simulink model "Piccolo_Induction_Motor(2)"  (R2022b)
settings: Solver=ode1  StartTime=0.0  StopTime=Inf  FixedStep=0.0001  RelTol=1e-3  EnableMultiTasking=on
PostLoadFcn:
  | ,try, rti_mdl_postloadfcn(bdroot, 'UpdateModel', 320, 'rti1104'); catch, disp(lasterr); end,
undefined symbols (not defined in the file or in its folder): Down, GPTRIP1SEL, GPTRIP2SEL, Km, TZ1, TZ2, Up
libraries: c2802xlib x3, c2806xlib x2, simulink x1, rtilib1104 x1, Piccolo_Library x1, c280xlib x1
settings Model: ExtModeTrigDuration=8  Creator=sb35user  LastModifiedBy=carls
settings SolverCC: ZeroCrossAlgorithm=Non-adaptive  AlgebraicLoopSolver=TrustRegion
settings DataIOCC: LimitDataPoints=on  SaveFormat=Array  SignalLoggingSaveFormat=ModelDataLogs  ReturnWorkspaceOutputs=off
settings OptimizationCC: BlockReduction=off  DefaultUnderspecifiedDataType=single  EnhancedBackFolding=on  PassReuseOutputArgsAs=Individual arguments  ExpressionDepthLimit=2147483647  InitFltsAndDblsToZero=on  MaxStackSize=1024  OptimizeBlockOrder=speed  DifferentSizesBufferReuse=on  OptimizationCustomize=off  DenormalBehavior=FlushToZero  EfficientTunableParamExpr=on
settings DebuggingCC: UnderspecifiedInitializationDetection=Classic  MergeDetectMultiDrivingBlocksExec=none  SolverPrmCheckMsg=warning  ParameterTunabilityLossMsg=error  FcnCallInpInsideContextMsg=warning  UnconnectedInputMsg=warning  UnconnectedOutputMsg=warning  UnconnectedLineMsg=warning  StateNameClashWarn=warning  SFUnexpectedBacktrackingDiag=warning  SFNoUnconditionalDefaultTransitionDiag=warning  SFExecutionAtInitializationDiag=none  SFMachineParentedDataDiag=warning  ArithmeticOperatorsInVariantConditions=warning
settings HardwareCC: ProdBitPerChar=16  ProdBitPerInt=16  ProdBitPerPointer=32  ProdBitPerSizeT=32  ProdBitPerPtrDiffT=32  ProdLargestAtomicInteger=Integer  ProdLargestAtomicFloat=None  ProdWordSize=16  ProdLongLongMode=on  ProdHWDeviceType=Texas Instruments->C2000  TargetIntDivRoundTo=Zero  TargetEndianess=BigEndian
settings ModelReferenceCC: PropagateSignalLabelsOutOfModel=off
settings SFSimCC: MATLABDynamicMemAlloc=off
settings RTWCC: Description=Embedded Coder  SystemTargetFile=ert.tlc  HardwareBoard=TI Piccolo F28069M LaunchPad  TLCOptions=-aInlineSetEventsForThisBaseRateFcn=TLC_FALSE -aSuppressMultiTaskScheduler=TLC_FALSE -aRateBasedStepFcn=1  TemplateMakefile=ert_default_tmf  Toolchain=Texas Instruments Code Composer Studio (C2000)
settings CodeAppCC: ForceParamTrailComments=on  IgnoreCustomStorageClasses=off  OperatorAnnotations=on  SimulinkDataObjDesc=on  SFDataObjDesc=on  InsertBlockDesc=on
settings ERTTargetCC: CodeReplacementLibrary=TI C28x  SupportContinuousTime=on  ExtModeTransport=4  ExtModeStaticAlloc=on  ExtModeAutomaticAllocSize=off  ExtModeMexFile=ext_xcp  ExtModeIntrfLevel=Level2 - Open
settings ConfigComp: CovMetricSettings=dw  CovSaveCumulativeToWorkspaceVar=on  CovSaveSingleToWorkspaceVar=on

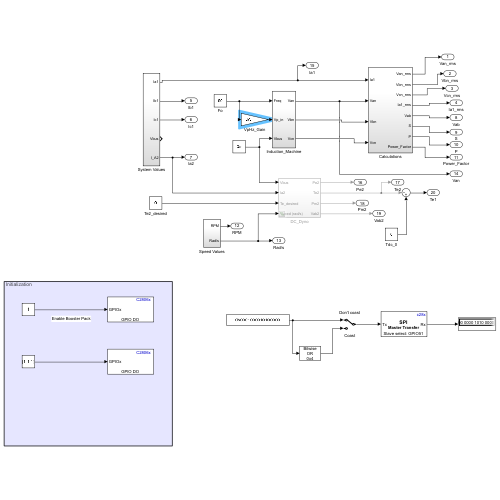
[thumbnail: Simulink's stored preview of the top-level diagram]
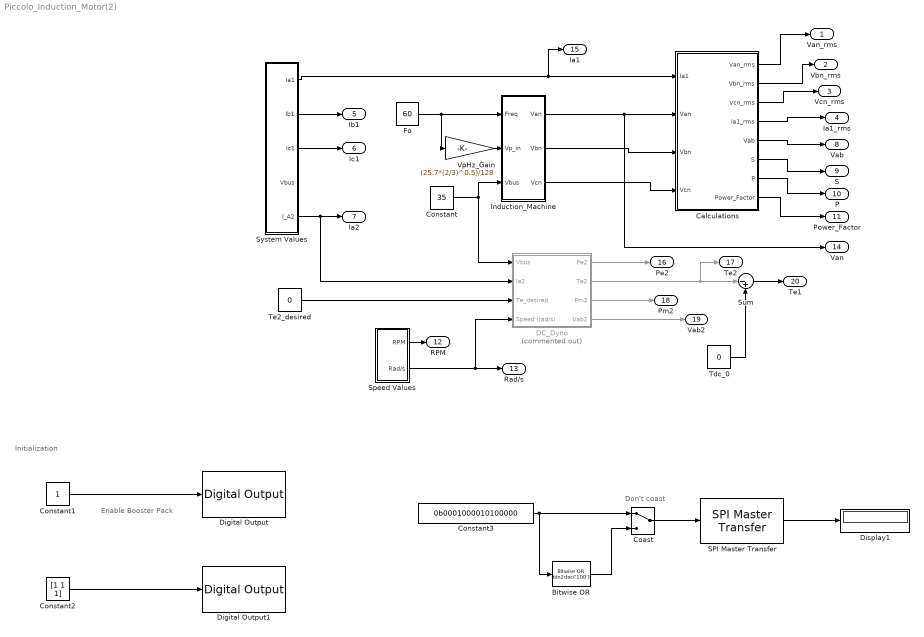
== system Piccolo_Induction_Motor(2) ==
  note: Don't coast
  note: Enable Booster Pack
  note: Initialization
  Bitwise OR : simulink/Logic and Bit Operations/Bitwise Operator  logicop=OR  UseBitMask=on  BitMask=bin2dec('100')  BitMaskRealWorld=Stored Integer
      settings: LibrarySourceBlock=|
      | simulink/Quick Insert/Logic and Bit
      | Operations/Bitwise OR
  Calculations : Subsystem
  Coast : ManualSwitch
  Constant : Constant  Value=35
  Constant1 : Constant
  Constant2 : Constant  Value=[1 1 1]
  Constant3 : Constant  Value=0b0001000010100000
  DC_Dyno : Subsystem  Commented=on
  Digital Output : c2806xlib/Digital Output  GPIO_Number=GPIO8~GPIO15  GPIO_Bit0=off  GPIO_BIT0_Toggle=off  GPIO_Bit1=off  GPIO_BIT1_Toggle=off  GPIO_Bit2=off  GPIO_BIT2_Toggle=off  GPIO_Bit3=off  GPIO_BIT3_Toggle=off  GPIO_Bit4=on  GPIO_BIT4_Toggle=off  GPIO_Bit5=off  GPIO_BIT5_Toggle=off  GPIO_Bit6=off  GPIO_BIT6_Toggle=off  GPIO_Bit7=off  GPIO_BIT7_Toggle=off
  Digital Output1 : c2806xlib/Digital Output  GPIO_Number=GPIO0~GPIO7  GPIO_Bit0=off  GPIO_BIT0_Toggle=off  GPIO_Bit1=on  GPIO_BIT1_Toggle=off  GPIO_Bit2=off  GPIO_BIT2_Toggle=off  GPIO_Bit3=on  GPIO_BIT3_Toggle=off  GPIO_Bit4=off  GPIO_BIT4_Toggle=off  GPIO_Bit5=on  GPIO_BIT5_Toggle=off  GPIO_Bit6=off  GPIO_BIT6_Toggle=off  GPIO_Bit7=off  GPIO_BIT7_Toggle=off
  Display1 : Display
      settings: Format=binary (Stored Integer)
  Fo : Constant  Value=60
  Induction_Machine : Subsystem
  SPI Master Transfer : c280xlib/SPI Master Transfer  SPISelect=SPI_A  ClockPolarity=Rising_edge  ClockPhase=No_delay  SPIModule=uint32(0)  Mode=Master  BusSpeed=uint32(1000000)  FirstBitToTransfer=Most significant bit (MSB)  ClockMode=0  BlockFunction=Transfer  EnableRegisterAddress=off  RegisterAddress=0  OutputDataType=int8  OutputDataLength=1  DataBits=16  UseCustomSSPin=Explicit GPIO calls  ActiveLowSSPin=Active low  Pin=51
      settings: LibrarySourceBlock=c2806xlib/SPI Master Transfer
  Speed Values : Subsystem
  Sum : Sum  Inputs=|-+
  System Values : Subsystem
  Tdc_0 : Constant  Value=0
  Te2_desired : Constant  Value=0
  VpHz_Gain : Gain  Gain=(25.7*(2/3)^0.5)/128
  Van_rms : Outport
  Vbn_rms : Outport  Port=2
  Vcn_rms : Outport  Port=3
  Ia1_rms : Outport  Port=4
  Ib1 : Outport  Port=5
  Ic1 : Outport  Port=6
  Ia2 : Outport  Port=7
  Vab : Outport  Port=8
  S : Outport  Port=9
  P : Outport  Port=10
  Power_Factor : Outport  Port=11
  RPM : Outport  Port=12
  Rad/s : Outport  Port=13
  Van : Outport  Port=14
  Ia1 : Outport  Port=15
  Pe2 : Outport  Port=16
  Te2 : Outport  Port=17
  Pm2 : Outport  Port=18
  Vab2 : Outport  Port=19
  Te1 : Outport  Port=20
  wires:
  System Values/2(Ib1) -> Ib1/1
  System Values/3(Ic1) -> Ic1/1
  Fo/1 -> Induction_Machine/1(Freq), VpHz_Gain/1
  VpHz_Gain/1 -> Induction_Machine/2(Vp_in)
  System Values/5(I_A2) -> Ia2/1, DC_Dyno/2(Ia2)
  Induction_Machine/3(Vcn) -> Calculations/4(Vcn)
  System Values/1(Ia1) -> Calculations/1(Ia1), Ia1/1
  Induction_Machine/1(Van) -> Calculations/2(Van), Van/1
  Induction_Machine/2(Vbn) -> Calculations/3(Vbn)
  Calculations/1(Van_rms) -> Van_rms/1
  Calculations/2(Vbn_rms) -> Vbn_rms/1
  Calculations/3(Vcn_rms) -> Vcn_rms/1
  Calculations/4(Ia1_rms) -> Ia1_rms/1
  Calculations/5(Vab) -> Vab/1
  Calculations/6(S) -> S/1
  Calculations/7(P) -> P/1
  Calculations/8(Power_Factor) -> Power_Factor/1
  Speed Values/1(RPM) -> RPM/1
  Speed Values/2(Rad/s) -> Rad/s/1, DC_Dyno/4(Speed (rad/s))
  Te2_desired/1 -> DC_Dyno/3(Te_desired)
  DC_Dyno/1(Pe2) -> Pe2/1
  DC_Dyno/3(Pm2) -> Pm2/1
  DC_Dyno/4(Vab2) -> Vab2/1
  DC_Dyno/2(Te2) -> Sum/1, Te2/1
  Tdc_0/1 -> Sum/2
  Sum/1 -> Te1/1
  Constant/1 -> Induction_Machine/3(Vbus), DC_Dyno/1(Vbus)
  Constant1/1 -> Digital Output/1
  Constant2/1 -> Digital Output1/1
  SPI Master Transfer/1 -> Display1/1
  Constant3/1 -> Bitwise OR/1, Coast/1
  Coast/1 -> SPI Master Transfer/1
  Bitwise OR/1 -> Coast/2

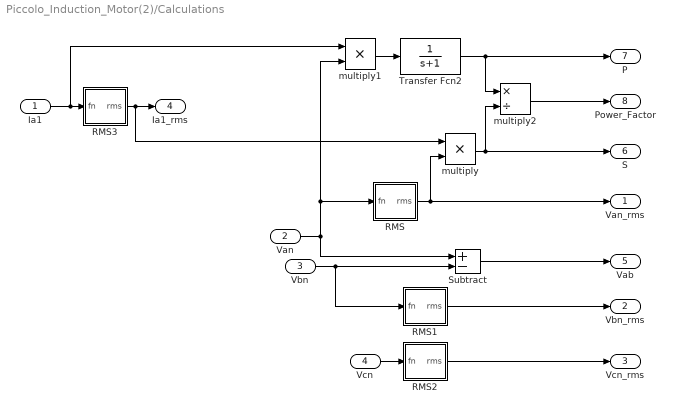
== system Piccolo_Induction_Motor(2)/Calculations ==
  Ia1 : Inport
  Van : Inport  Port=2
  Vbn : Inport  Port=3
  Vcn : Inport  Port=4
  RMS : Subsystem
  RMS1 : Subsystem
  RMS2 : Subsystem
  RMS3 : Subsystem
  Subtract : Sum  Inputs=+-
  Transfer Fcn2 : TransferFcn  Denominator=[1 1]
  multiply : Product  Inputs=**
  multiply1 : Product  Inputs=**
  multiply2 : Product  Inputs=*/
  Van_rms : Outport
  Vbn_rms : Outport  Port=2
  Vcn_rms : Outport  Port=3
  Ia1_rms : Outport  Port=4
  Vab : Outport  Port=5
  S : Outport  Port=6
  P : Outport  Port=7
  Power_Factor : Outport  Port=8
  wires:
  Subtract/1 -> Vab/1
  Van/1 -> multiply1/2, RMS/1(fn), Subtract/1
  Vbn/1 -> RMS1/1(fn), Subtract/2
  RMS/1(rms) -> Van_rms/1, multiply/2
  RMS1/1(rms) -> Vbn_rms/1
  RMS2/1(rms) -> Vcn_rms/1
  Ia1/1 -> multiply1/1, RMS3/1(fn)
  RMS3/1(rms) -> Ia1_rms/1, multiply/1
  multiply/1 -> S/1, multiply2/2
  Transfer Fcn2/1 -> P/1, multiply2/1
  multiply1/1 -> Transfer Fcn2/1
  multiply2/1 -> Power_Factor/1
  Vcn/1 -> RMS2/1(fn)

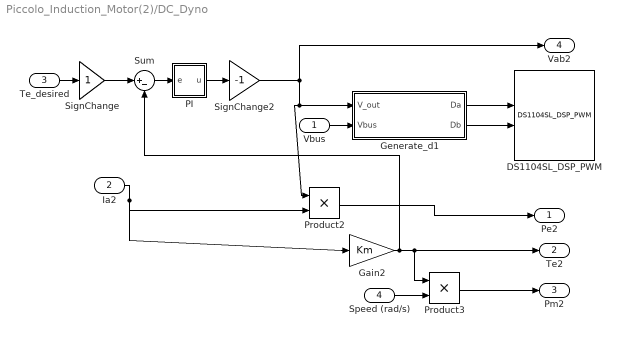
== system Piccolo_Induction_Motor(2)/DC_Dyno ==
  Vbus : Inport
  Ia2 : Inport  Port=2
  Te_desired : Inport  Port=3
  Speed (rad/s) : Inport  Port=4
  DS1104SL_DSP_PWM : rtilib1104/DS1104 SLAVE DSP/DS1104SL_DSP_PWM  SystemSampleTime=-1  Parameters=[]  TDef=[]  BoardType=[]  PwmMode=[]  Frequency=[]  InitValue=[]  TermMode=[]  TermValue=[]  Polarity=[]  DialogFcn=[]  Reserved1=[]  Reserved2=[]  Reserved3=[]  Reserved4=[]  Revision=[]  UnitName=[]  UnitValues=[]  DSProperties=struct('RTI',struct('Version',uint32(2),'BlockType',struct('isSLSource',uint8(0),'isSLSink',uint8(1),'isHWSource',uint8(0),'isHWSink',uint8(1),'isSetup',uint8(0),'isInline',uint8(1),'isNonInline',uint8(0),'isInterrupt',uint8(0),'isChannelwise',uint8(0)),'IOBoardType','DS1104SLAVE','UnitType','PWM','Identifier','PWM','DialogType','ML','BlockSet','NONE','SlaveProcessor','F240'))  RTIBlockInterface=struct('InputPortsActive',[1 1 1 1],'InputPortsWidth',int32([1 1 1 1]),'InputPortsName',{{['PWM Channel 1'],['PWM Channel 2'],['PWM Channel 3'],['PWM Channel 4']}},'IWork',{{{'',uint32(4)}}},'DialogFcn','rti1104slavepwmgui','InitLevel',1,'BlockDisplay',{{'','auto'}},'IconTransparency','on','MultiSFcn',4,'BlockName',struct('Token',{{'DS1104SL_DSP_PWM'}}))  RTIBlockParameters=struct('PWMSymmetryMode',{{1,'OFF',[]}},'PWMFrequency',{{'10000','OFF',[]}},'PWMPolarityMode',{{[1 1 1 1 1],'OFF',[]}},'ChannelNo',{{[1 2 3 4],'OFF',[]}},'SuspendModeInit',{{[1 1 1 1 1],'OFF',[]}},'TTLModeInit',{{[2 2 2 2 2],'OFF',[]}},'DutyCycleInitValueCh1',{{'0.5','OFF',[]}},'DutyCycleInitValueCh2',{{'0.5','OFF',[]}},'DutyCycleInitValueCh3',{{'0.5','OFF',[]}},'DutyCycleInitValueCh4',{{'0.5','OFF',[]}},'DutyCycleInitValueCh5',{{'0.5','OFF',[]}},'EnablePWMStop',{{[0 0 0 0 0],'OFF',[]}},'SuspendModeTerm',{{[1 1 1 1 1],'OFF',[]}},'TTLModeTerm',{{[2 2 2 2 2],'OFF',[]}},'DutyCycleTermValueCh1',{{'0.5','OFF',[]}},'DutyCycleTermValueCh2',{{'0.5','OFF',[]}},'DutyCycleTermValueCh3',{{'0.5','OFF',[]}},'DutyCycleTermValueCh4',{{'0.5','OFF',[]}},'DutyCycleTermValueCh5',{{'0.5','OFF',[]}},'TLCFileName',{{'rti1104pwm','OFF',[]}})  RTISFcnParameters=struct('PWMSymmetryMode','double','PWMFrequency','double','PWMPolarityMode','double','ChannelNo','double','SuspendModeInit','double','TTLModeInit','double','DutyCycleInitValueCh1','double','DutyCycleInitValueCh2','double','DutyCycleInitValueCh3','double','DutyCycleInitValueCh4','double','EnablePWMStop','double','SuspendModeTerm','double','TTLModeTerm','double','DutyCycleTermValueCh1','double','DutyCycleTermValueCh2','double','DutyCycleTermValueCh3','double','DutyCycleTermValueCh4','double','TLCFileName','char')  RTIBlockParaDefault=struct('PWMSymmetryMode',1,'PWMFrequency',100,'PWMPolarityMode',[1 1 1 1 1],'ChannelNo',[1 2 3 4],'SuspendModeInit',[1 1 1 1 1],'TTLModeInit',[2 2 2 2 2],'DutyCycleInitValueCh1',0.5,'DutyCycleInitValueCh2',0.5,'DutyCycleInitValueCh3',0.5,'DutyCycleInitValueCh4',0.5,'DutyCycleInitValueCh5',0.5,'EnablePWMStop',[1 1 1 1 0],'SuspendModeTerm',[1 1 1 1 1],'TTLModeTerm',[2 2 2 2 2],'DutyCycleTermValueCh1',0.5,'DutyCycleTermValueCh2',0.5,'DutyCycleTermValueCh3',0.5,'DutyCycleTermValueCh4',0.5,'DutyCycleTermValueCh5',0.5,'TLCFileName','rti1104pwm')
  Gain2 : Gain  Gain=Km
  Generate_d1 : Subsystem
  PI : Subsystem
  Product2 : Product  RndMeth=Zero
  Product3 : Product  RndMeth=Zero
  SignChange : Gain
  SignChange2 : Gain  Gain=-1
  Sum : Sum  Inputs=|+-
  Pe2 : Outport
  Te2 : Outport  Port=2
  Pm2 : Outport  Port=3
  Vab2 : Outport  Port=4
  wires:
  PI/1(u) -> SignChange2/1
  Generate_d1/1(Da) -> DS1104SL_DSP_PWM/2
  Generate_d1/2(Db) -> DS1104SL_DSP_PWM/3
  Product2/1 -> Pe2/1
  Product3/1 -> Pm2/1
  Sum/1 -> PI/1(e)
  Gain2/1 -> Sum/2, Te2/1, Product3/1
  Vbus/1 -> Generate_d1/2(Vbus)
  Ia2/1 -> Product2/2, Gain2/1
  Speed (rad/s)/1 -> Product3/2
  Te_desired/1 -> SignChange/1
  SignChange/1 -> Sum/1
  SignChange2/1 -> Product2/1, Generate_d1/1(V_out), Vab2/1

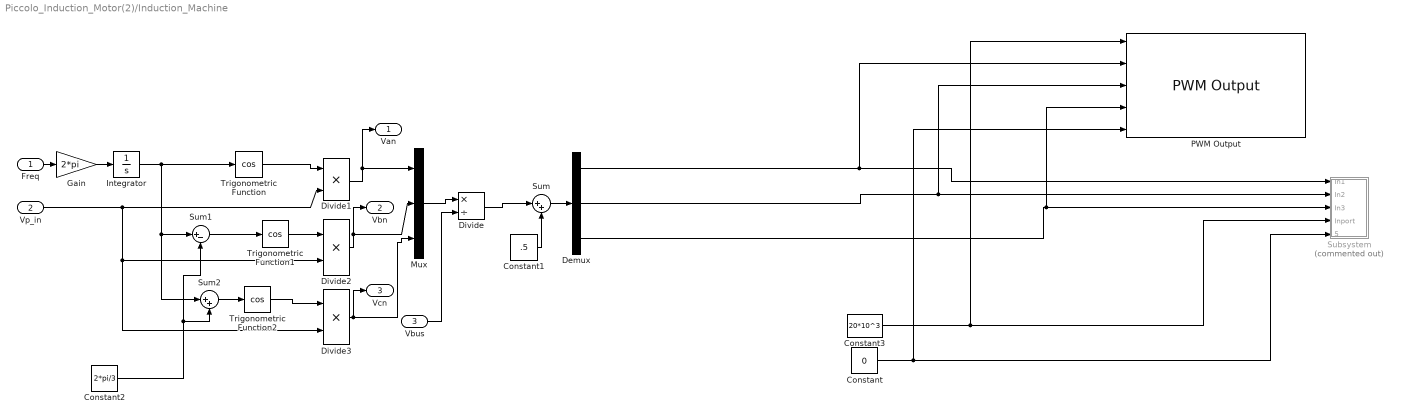
== system Piccolo_Induction_Motor(2)/Induction_Machine ==
  Freq : Inport
  Vp_in : Inport  Port=2
  Vbus : Inport  Port=3
  Constant : Constant  Value=0
  Constant1 : Constant  Value=.5
  Constant2 : Constant  Value=2*pi/3
  Constant3 : Constant  Value=20*10^3
  Demux : Demux  Outputs=3
  Divide : Product  Inputs=*/
  Divide1 : Product  Inputs=**
  Divide2 : Product  Inputs=**
  Divide3 : Product  Inputs=**
  Gain : Gain  Gain=2*pi
  Integrator : Integrator
  Mux : Mux  Inputs=3
  PWM Output : Piccolo_Library/PWM Output  Pack=1  Prescale=1
      settings: SourceProductName=Piccolo Motor Control
  Subsystem : Subsystem  Commented=on
  Sum : Sum  Inputs=|++
  Sum1 : Sum  Inputs=|+-
  Sum2 : Sum  Inputs=|++
  Trigonometric Function : Trigonometry  Operator=cos
  Trigonometric Function1 : Trigonometry  Operator=cos
  Trigonometric Function2 : Trigonometry  Operator=cos
  Van : Outport
  Vbn : Outport  Port=2
  Vcn : Outport  Port=3
  wires:
  Constant1/1 -> Sum/2
  Sum/1 -> Demux/1
  Mux/1 -> Divide/1
  Divide/1 -> Sum/1
  Vbus/1 -> Divide/2
  Gain/1 -> Integrator/1
  Freq/1 -> Gain/1
  Integrator/1 -> Trigonometric Function/1, Sum2/1, Sum1/1
  Trigonometric Function/1 -> Divide1/1
  Vp_in/1 -> Divide1/2, Divide2/2, Divide3/2
  Divide1/1 -> Mux/1, Van/1
  Sum1/1 -> Trigonometric Function1/1
  Divide2/1 -> Mux/2, Vbn/1
  Trigonometric Function1/1 -> Divide2/1
  Constant2/1 -> Sum1/2, Sum2/2
  Sum2/1 -> Trigonometric Function2/1
  Trigonometric Function2/1 -> Divide3/1
  Divide3/1 -> Mux/3, Vcn/1
  Demux/1 -> PWM Output/2, Subsystem/1(In1)
  Demux/2 -> PWM Output/3, Subsystem/2(In2)
  Demux/3 -> PWM Output/4, Subsystem/3(In3)
  Constant/1 -> PWM Output/5, Subsystem/5(Inport1)
  Constant3/1 -> PWM Output/1, Subsystem/4(Inport)

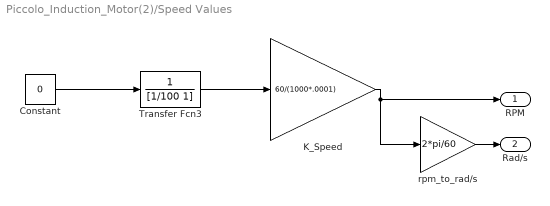
== system Piccolo_Induction_Motor(2)/Speed Values ==
  Constant : Constant  Value=0
  K_Speed : Gain  Gain=60/(1000*.0001)
  Transfer Fcn3 : TransferFcn  Denominator=[1/100 1]
  rpm_to_rad/s : Gain  Gain=2*pi/60
  RPM : Outport
  Rad/s : Outport  Port=2
  wires:
  K_Speed/1 -> rpm_to_rad/s/1, RPM/1
  rpm_to_rad/s/1 -> Rad/s/1
  Constant/1 -> Transfer Fcn3/1
  Transfer Fcn3/1 -> K_Speed/1

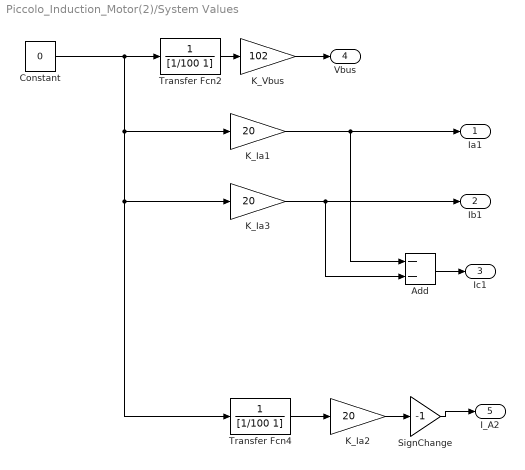
== system Piccolo_Induction_Motor(2)/System Values ==
  Add : Sum  Inputs=--
  Constant : Constant  Value=0
  K_Ia1 : Gain  Gain=20
  K_Ia2 : Gain  Gain=20
  K_Ia3 : Gain  Gain=20
  K_Vbus : Gain  Gain=102
  SignChange : Gain  Gain=-1
  Transfer Fcn2 : TransferFcn  Denominator=[1/100 1]
  Transfer Fcn4 : TransferFcn  Denominator=[1/100 1]
  Ia1 : Outport
  Ib1 : Outport  Port=2
  Ic1 : Outport  Port=3
  Vbus : Outport  Port=4
  I_A2 : Outport  Port=5
  wires:
  Transfer Fcn4/1 -> K_Ia2/1
  Constant/1 -> Transfer Fcn4/1, K_Ia3/1, K_Ia1/1, Transfer Fcn2/1
  K_Ia2/1 -> SignChange/1
  Transfer Fcn2/1 -> K_Vbus/1
  K_Ia1/1 -> Ia1/1, Add/1
  K_Vbus/1 -> Vbus/1
  K_Ia3/1 -> Ib1/1, Add/2
  Add/1 -> Ic1/1
  SignChange/1 -> I_A2/1

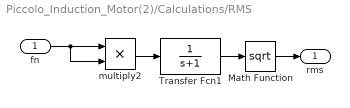
== system Piccolo_Induction_Motor(2)/Calculations/RMS ==
  fn : Inport
  Math Function : Math  Operator=sqrt  SignedPower=on
  Transfer Fcn1 : TransferFcn  Denominator=[1 1]
  multiply2 : Product  Inputs=**
  rms : Outport
  wires:
  multiply2/1 -> Transfer Fcn1/1
  Transfer Fcn1/1 -> Math Function/1
  fn/1 -> multiply2/1, multiply2/2
  Math Function/1 -> rms/1

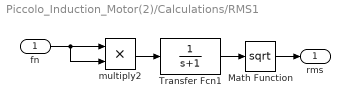
== system Piccolo_Induction_Motor(2)/Calculations/RMS1 ==
  fn : Inport
  Math Function : Math  Operator=sqrt  SignedPower=on
  Transfer Fcn1 : TransferFcn  Denominator=[1 1]
  multiply2 : Product  Inputs=**
  rms : Outport
  wires:
  Math Function/1 -> rms/1
  fn/1 -> multiply2/2, multiply2/1
  Transfer Fcn1/1 -> Math Function/1
  multiply2/1 -> Transfer Fcn1/1

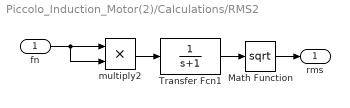
== system Piccolo_Induction_Motor(2)/Calculations/RMS2 ==
  fn : Inport
  Math Function : Math  Operator=sqrt  SignedPower=on
  Transfer Fcn1 : TransferFcn  Denominator=[1 1]
  multiply2 : Product  Inputs=**
  rms : Outport
  wires:
  multiply2/1 -> Transfer Fcn1/1
  Transfer Fcn1/1 -> Math Function/1
  fn/1 -> multiply2/1, multiply2/2
  Math Function/1 -> rms/1

== system Piccolo_Induction_Motor(2)/Calculations/RMS3 ==
  fn : Inport
  Math Function : Math  Operator=sqrt  SignedPower=on
  Transfer Fcn1 : TransferFcn  Denominator=[1 1]
  multiply2 : Product  Inputs=**
  rms : Outport
  wires:
  Math Function/1 -> rms/1
  fn/1 -> multiply2/2, multiply2/1
  Transfer Fcn1/1 -> Math Function/1
  multiply2/1 -> Transfer Fcn1/1

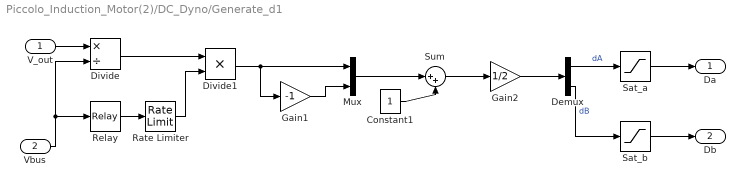
== system Piccolo_Induction_Motor(2)/DC_Dyno/Generate_d1 ==
  V_out : Inport
  Vbus : Inport  Port=2
  Constant1 : Constant
  Demux : Demux  Outputs=2
  Divide : Product  Inputs=*/
  Divide1 : Product  Inputs=**
  Gain1 : Gain  Gain=-1
  Gain2 : Gain  Gain=1/2
  Mux : Mux  Inputs=2
  Rate Limiter : RateLimiter  RisingSlewLimit=.7  SampleTimeMode=inherited
  Relay : Relay  OnSwitchValue=10  OffSwitchValue=10
  Sat_a : Saturate  UpperLimit=.98  LowerLimit=0
  Sat_b : Saturate  UpperLimit=.98  LowerLimit=0
  Sum : Sum  Inputs=|++
  Da : Outport
  Db : Outport  Port=2
  wires:
  Divide1/1 -> Gain1/1, Mux/1
  Rate Limiter/1 -> Divide1/2
  Divide/1 -> Divide1/1
  Relay/1 -> Rate Limiter/1
  Sat_b/1 -> Db/1
  Sat_a/1 -> Da/1
  Demux/2 -> Sat_b/1  "dB"
  Vbus/1 -> Relay/1, Divide/2
  Demux/1 -> Sat_a/1  "dA"
  V_out/1 -> Divide/1
  Gain2/1 -> Demux/1
  Sum/1 -> Gain2/1
  Gain1/1 -> Mux/2
  Mux/1 -> Sum/1
  Constant1/1 -> Sum/2

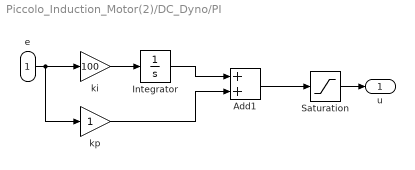
== system Piccolo_Induction_Motor(2)/DC_Dyno/PI ==
  e : Inport
  Add1 : Sum
  Integrator : Integrator  LimitOutput=on  UpperSaturationLimit=42  LowerSaturationLimit=-42
  Saturation : Saturate  UpperLimit=42  LowerLimit=-42
  ki : Gain  Gain=100
  kp : Gain
  u : Outport
  wires:
  e/1 -> kp/1, ki/1
  Add1/1 -> Saturation/1
  kp/1 -> Add1/2
  Integrator/1 -> Add1/1
  ki/1 -> Integrator/1
  Saturation/1 -> u/1

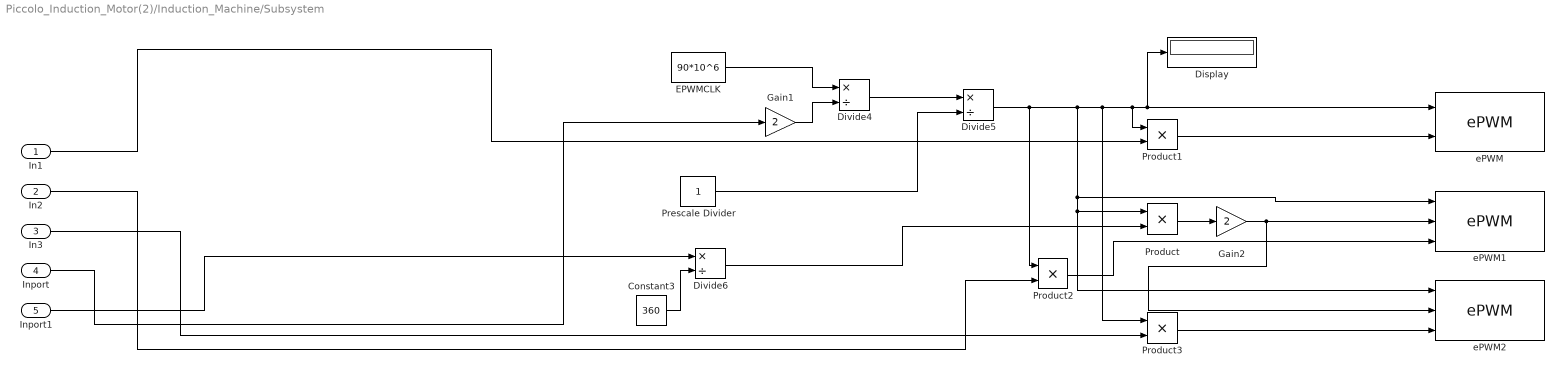
== system Piccolo_Induction_Motor(2)/Induction_Machine/Subsystem ==
  In1 : Inport
  In2 : Inport  Port=2
  In3 : Inport  Port=3
  Inport : Inport  Port=4
  Inport1 : Inport  Port=5
  Constant3 : Constant  Value=360
  Display : Display
  Divide4 : Product  Inputs=*/
  Divide5 : Product  Inputs=*/
  Divide6 : Product  Inputs=*/
  EPWMCLK : Constant  Value=90*10^6
  Gain1 : Gain  Gain=2
  Gain2 : Gain  Gain=2
  Prescale Divider : Constant
  Product{,1..3} (4 alike) : Product
  ePWM : c2802xlib/ePWM  PwmType=C2000  useModule=ePWM1  ePWMxLINKTBPRD=Not Linked  periodUnits=Clock cycles  timerSource=Input port  timerPeriod_clk=64000  timerPeriod_sec=0.0001  tbshadow=Counter equals to zero  countingMode=Up-Down  phaseActiveEnable=Disable  phaseDirection=Count down after sync  phaseActive=0  synchronizationEnable=off  dcaevt1Sync=off  dcbevt1Sync=off  synchronizationOption=Counter equals to zero (CTR=Zero)  dcbevt1SyncOut=off  dcaevt1SyncOut=off  cmpdSyncOut=off  cmpcSyncOut=off  cmpbSyncOut=off  zeroSyncOut=off  swfSyncOut=off  perSynchronizationOption=Counter equals to period (CTR=PRD)  clockPrescale=1  HSclockPrescale=1  enswap=off  ePWMxAStatus=on  ePWMxAactionLogic1=Set  ePWMxAactionLogic2=Clear  ePWMxAactionLogic3=Clear  ePWMxAactionLogic4=Set  ePWMxAactionLogic5=Do nothing  ePWMxAactionLogic6=Do nothing  ePWMxACSFenable=off  ePWMxACSFvalue=Forcing disable  ePWMxASFreload=Zero  ePWMxBStatus=off  ePWMxBactionLogic1=Set  ePWMxBactionLogic2=Clear  ePWMxBactionLogic3=Do nothing  ePWMxBactionLogic4=Do nothing  ePWMxBactionLogic5=Clear  ePWMxBactionLogic6=Set  ePWMxBCSFenable=off  ePWMxBCSFvalue=Forcing disable  ePWMxBSFreload=Zero  ePWNxBOutWay=off  ePWMxLINKCMPA=Not Linked  CMPAUnits=Clock cycles  CMPASource=Input port  CMPAValue_per=50  CMPAValue_clk=32000  enCMPAshadow=Counter equals to zero (CTR=Zero)  ePWMxLINKCMPB=Not Linked  CMPBUnits=Clock cycles  CMPBSource=Specify via dialog  CMPBValue_per=50  CMPBValue_clk=32000  enCMPBshadow=Counter equals to zero (CTR=Zero)  ePWMxLINKCMPC=Not Linked  CMPCUnits=Clock cycles  CMPCSource=Specify via dialog  CMPCValue_per=50  CMPCValue_clk=32000  enCMPCshadow=Counter equals to zero (CTR=Zero)  ePWMxLINKCMPD=Not Linked  CMPDUnits=Clock cycles  CMPDSource=Specify via dialog  CMPDValue_per=50  CMPDValue_clk=32000  enCMPDshadow=Counter equals to zero (CTR=Zero)  enableDBePWMxA=off  enableDBePWMxB=off  enhalfcycle=off  DBpolarity=Active high (AH)  DBedgeDelay=Positive  DBSource_ePWMxA=ePWMxA  DBSource_ePWMxB=ePWMxA  DBPeriodUnits=Clock cycles  DBperiodSource=Specify via dialog  REDperiod=0  FEDperiod=0  REDperiod_sec=0  FEDperiod_sec=0  LoadModeDBRED=Immediate without using shadow  LoadModeDBFED=Immediate without using shadow  adcstartModuleA=off  adcrequestEventA=First event  adcstartEventA=Counter equals to zero (CTR=Zero)  adcstartEventA_type2=Digital Compare Module A Event 1 start of conversion (DCAEVT1.soc)  adcstartModuleB=off  adcrequestEventB=First event  adcstartEventB=Counter equals to zero (CTR=Zero)  adcstartEventB_type2=Counter equals to zero (CTR=Zero)  intEn=off  intPrd=First event  intSel=Counter equals to zero (CTR=Zero)  intSel_type2=Counter equals to zero (CTR=Zero)  hrpe=off  enHRPWM=off  HRPWM_LoadMode=Counter equals to period (CTR=PRD)  HRPWM_CTLMode=Duty or Period control mode  HRPWM_EDGMode=Both edge  hrpeb=off  enHRPWMB=off  HRPWM_LoadModeB=Counter equals to zero (CTR=ZERO)  HRPWM_CTLModeB=Duty or Period control mode  HRPWM_EDGModeB=Both edge  enHRDBRED=off  enHRDBFED=off  enSFO=on  enautoconv=on  chopperEnable=off  chopperFrequency=1  chopperFirstwidth=1  chopperDuty=12.5%  tripZonesource=Specify via dialog  tzselOSHT1=off  tzselOSHT2=off  tzselOSHT3=off  tzselOSHDCAEV1=off  tzselOSHDCBEV1=off  tzselCBC1=off  tzselCBC2=off  tzselCBC3=off  tzselCBCDCAEV2=off  tzselCBCDCBEV2=off  tzselOSHT4=off  tzselOSHT5=off  tzselOSHT6=off  tzselCBC4=off  tzselCBC5=off  tzselCBC6=off  enTzOstIntr=off  enTzCbcIntr=off  enTzDCAEVT1Intr=off  enTzDCAEVT2Intr=off  enTzDCBEVT1Intr=off  enTzDCBEVT2Intr=off  ePWMxAforced=No action  ePWMxBforced=No action  DCAEVT1forced=No action  DCBEVT1forced=No action  DCAEVT2forced=No action  DCBEVT2forced=No action  dcah=Trip Zone 1 input (TZ1)  dcal=Trip Zone 1 input (TZ1)  dcbh=Trip Zone 1 input (TZ1)  dcbl=Trip Zone 1 input (TZ1)  dcah_type2=GPTRIP1SEL/(TZ1)  dcal_type2=GPTRIP2SEL/(TZ2)  dcbh_type2=GPTRIP1SEL/(TZ1)  dcbl_type2=GPTRIP2SEL/(TZ2)  gendcaevt1=Event disabled  gendcaevt2=Event disabled  gendcbevt1=Event disabled  gendcbevt2=Event disabled  dcaevt1src=DCAEVT1 with sync  dcaevt2src=DCAEVT2 with sync  dcbevt1src=DCBEVT1 with sync  dcbevt2src=DCBEVT2 with sync  pulsesel=Counter equals to zero (CTR=Zero)  blankinv=off  blankoffset=0  blankwidth=0  evsrcsel=Filtered version of DCAEVT1 (DCAEVT1FILT)  encape=off
      settings: LibrarySourceBlock=c2806xlib/ePWM
  ePWM1 : c2802xlib/ePWM  PwmType=C2000  useModule=ePWM2  ePWMxLINKTBPRD=Not Linked  periodUnits=Clock cycles  timerSource=Input port  timerPeriod_clk=64000  timerPeriod_sec=0.0001  tbshadow=Counter equals to zero  countingMode=Up-Down  phaseActiveEnable=Set counter to phase value specified via input port  phaseDirection=Count down after sync  phaseActive=0  synchronizationEnable=off  dcaevt1Sync=off  dcbevt1Sync=off  synchronizationOption=Counter equals to zero (CTR=Zero)  dcbevt1SyncOut=off  dcaevt1SyncOut=off  cmpdSyncOut=off  cmpcSyncOut=off  cmpbSyncOut=off  zeroSyncOut=off  swfSyncOut=off  perSynchronizationOption=Counter equals to period (CTR=PRD)  clockPrescale=1  HSclockPrescale=1  enswap=off  ePWMxAStatus=on  ePWMxAactionLogic1=Set  ePWMxAactionLogic2=Clear  ePWMxAactionLogic3=Clear  ePWMxAactionLogic4=Set  ePWMxAactionLogic5=Do nothing  ePWMxAactionLogic6=Do nothing  ePWMxACSFenable=off  ePWMxACSFvalue=Forcing disable  ePWMxASFreload=Zero  ePWMxBStatus=off  ePWMxBactionLogic1=Set  ePWMxBactionLogic2=Clear  ePWMxBactionLogic3=Do nothing  ePWMxBactionLogic4=Do nothing  ePWMxBactionLogic5=Clear  ePWMxBactionLogic6=Set  ePWMxBCSFenable=off  ePWMxBCSFvalue=Forcing disable  ePWMxBSFreload=Zero  ePWNxBOutWay=off  ePWMxLINKCMPA=Not Linked  CMPAUnits=Clock cycles  CMPASource=Input port  CMPAValue_per=50  CMPAValue_clk=32000  enCMPAshadow=Counter equals to zero (CTR=Zero)  ePWMxLINKCMPB=Not Linked  CMPBUnits=Clock cycles  CMPBSource=Specify via dialog  CMPBValue_per=50  CMPBValue_clk=32000  enCMPBshadow=Counter equals to zero (CTR=Zero)  ePWMxLINKCMPC=Not Linked  CMPCUnits=Clock cycles  CMPCSource=Specify via dialog  CMPCValue_per=50  CMPCValue_clk=32000  enCMPCshadow=Counter equals to zero (CTR=Zero)  ePWMxLINKCMPD=Not Linked  CMPDUnits=Clock cycles  CMPDSource=Specify via dialog  CMPDValue_per=50  CMPDValue_clk=32000  enCMPDshadow=Counter equals to zero (CTR=Zero)  enableDBePWMxA=off  enableDBePWMxB=off  enhalfcycle=off  DBpolarity=Active high (AH)  DBedgeDelay=Positive  DBSource_ePWMxA=ePWMxA  DBSource_ePWMxB=ePWMxA  DBPeriodUnits=Clock cycles  DBperiodSource=Specify via dialog  REDperiod=0  FEDperiod=0  REDperiod_sec=0  FEDperiod_sec=0  LoadModeDBRED=Immediate without using shadow  LoadModeDBFED=Immediate without using shadow  adcstartModuleA=off  adcrequestEventA=First event  adcstartEventA=Counter equals to zero (CTR=Zero)  adcstartEventA_type2=Digital Compare Module A Event 1 start of conversion (DCAEVT1.soc)  adcstartModuleB=off  adcrequestEventB=First event  adcstartEventB=Counter equals to zero (CTR=Zero)  adcstartEventB_type2=Counter equals to zero (CTR=Zero)  intEn=off  intPrd=First event  intSel=Counter equals to zero (CTR=Zero)  intSel_type2=Counter equals to zero (CTR=Zero)  hrpe=off  enHRPWM=off  HRPWM_LoadMode=Counter equals to period (CTR=PRD)  HRPWM_CTLMode=Duty or Period control mode  HRPWM_EDGMode=Both edge  hrpeb=off  enHRPWMB=off  HRPWM_LoadModeB=Counter equals to zero (CTR=ZERO)  HRPWM_CTLModeB=Duty or Period control mode  HRPWM_EDGModeB=Both edge  enHRDBRED=off  enHRDBFED=off  enSFO=on  enautoconv=on  chopperEnable=off  chopperFrequency=1  chopperFirstwidth=1  chopperDuty=12.5%  tripZonesource=Specify via dialog  tzselOSHT1=off  tzselOSHT2=off  tzselOSHT3=off  tzselOSHDCAEV1=off  tzselOSHDCBEV1=off  tzselCBC1=off  tzselCBC2=off  tzselCBC3=off  tzselCBCDCAEV2=off  tzselCBCDCBEV2=off  tzselOSHT4=off  tzselOSHT5=off  tzselOSHT6=off  tzselCBC4=off  tzselCBC5=off  tzselCBC6=off  enTzOstIntr=off  enTzCbcIntr=off  enTzDCAEVT1Intr=off  enTzDCAEVT2Intr=off  enTzDCBEVT1Intr=off  enTzDCBEVT2Intr=off  ePWMxAforced=No action  ePWMxBforced=No action  DCAEVT1forced=No action  DCBEVT1forced=No action  DCAEVT2forced=No action  DCBEVT2forced=No action  dcah=Trip Zone 1 input (TZ1)  dcal=Trip Zone 1 input (TZ1)  dcbh=Trip Zone 1 input (TZ1)  dcbl=Trip Zone 1 input (TZ1)  dcah_type2=GPTRIP1SEL/(TZ1)  dcal_type2=GPTRIP2SEL/(TZ2)  dcbh_type2=GPTRIP1SEL/(TZ1)  dcbl_type2=GPTRIP2SEL/(TZ2)  gendcaevt1=Event disabled  gendcaevt2=Event disabled  gendcbevt1=Event disabled  gendcbevt2=Event disabled  dcaevt1src=DCAEVT1 with sync  dcaevt2src=DCAEVT2 with sync  dcbevt1src=DCBEVT1 with sync  dcbevt2src=DCBEVT2 with sync  pulsesel=Counter equals to zero (CTR=Zero)  blankinv=off  blankoffset=0  blankwidth=0  evsrcsel=Filtered version of DCAEVT1 (DCAEVT1FILT)  encape=off
      settings: LibrarySourceBlock=c2806xlib/ePWM
  ePWM2 : c2802xlib/ePWM  PwmType=C2000  useModule=ePWM3  ePWMxLINKTBPRD=Not Linked  periodUnits=Clock cycles  timerSource=Input port  timerPeriod_clk=64000  timerPeriod_sec=0.0001  tbshadow=Counter equals to zero  countingMode=Up-Down  phaseActiveEnable=Set counter to phase value specified via input port  phaseDirection=Count down after sync  phaseActive=0  synchronizationEnable=off  dcaevt1Sync=off  dcbevt1Sync=off  synchronizationOption=Counter equals to zero (CTR=Zero)  dcbevt1SyncOut=off  dcaevt1SyncOut=off  cmpdSyncOut=off  cmpcSyncOut=off  cmpbSyncOut=off  zeroSyncOut=off  swfSyncOut=off  perSynchronizationOption=Counter equals to period (CTR=PRD)  clockPrescale=1  HSclockPrescale=1  enswap=off  ePWMxAStatus=on  ePWMxAactionLogic1=Set  ePWMxAactionLogic2=Clear  ePWMxAactionLogic3=Clear  ePWMxAactionLogic4=Set  ePWMxAactionLogic5=Do nothing  ePWMxAactionLogic6=Do nothing  ePWMxACSFenable=off  ePWMxACSFvalue=Forcing disable  ePWMxASFreload=Zero  ePWMxBStatus=off  ePWMxBactionLogic1=Set  ePWMxBactionLogic2=Clear  ePWMxBactionLogic3=Do nothing  ePWMxBactionLogic4=Do nothing  ePWMxBactionLogic5=Clear  ePWMxBactionLogic6=Set  ePWMxBCSFenable=off  ePWMxBCSFvalue=Forcing disable  ePWMxBSFreload=Zero  ePWNxBOutWay=off  ePWMxLINKCMPA=Not Linked  CMPAUnits=Clock cycles  CMPASource=Input port  CMPAValue_per=50  CMPAValue_clk=32000  enCMPAshadow=Counter equals to zero (CTR=Zero)  ePWMxLINKCMPB=Not Linked  CMPBUnits=Clock cycles  CMPBSource=Specify via dialog  CMPBValue_per=50  CMPBValue_clk=32000  enCMPBshadow=Counter equals to zero (CTR=Zero)  ePWMxLINKCMPC=Not Linked  CMPCUnits=Clock cycles  CMPCSource=Specify via dialog  CMPCValue_per=50  CMPCValue_clk=32000  enCMPCshadow=Counter equals to zero (CTR=Zero)  ePWMxLINKCMPD=Not Linked  CMPDUnits=Clock cycles  CMPDSource=Specify via dialog  CMPDValue_per=50  CMPDValue_clk=32000  enCMPDshadow=Counter equals to zero (CTR=Zero)  enableDBePWMxA=off  enableDBePWMxB=off  enhalfcycle=off  DBpolarity=Active high (AH)  DBedgeDelay=Positive  DBSource_ePWMxA=ePWMxA  DBSource_ePWMxB=ePWMxA  DBPeriodUnits=Clock cycles  DBperiodSource=Specify via dialog  REDperiod=0  FEDperiod=0  REDperiod_sec=0  FEDperiod_sec=0  LoadModeDBRED=Immediate without using shadow  LoadModeDBFED=Immediate without using shadow  adcstartModuleA=off  adcrequestEventA=First event  adcstartEventA=Counter equals to zero (CTR=Zero)  adcstartEventA_type2=Digital Compare Module A Event 1 start of conversion (DCAEVT1.soc)  adcstartModuleB=off  adcrequestEventB=First event  adcstartEventB=Counter equals to zero (CTR=Zero)  adcstartEventB_type2=Counter equals to zero (CTR=Zero)  intEn=off  intPrd=First event  intSel=Counter equals to zero (CTR=Zero)  intSel_type2=Counter equals to zero (CTR=Zero)  hrpe=off  enHRPWM=off  HRPWM_LoadMode=Counter equals to period (CTR=PRD)  HRPWM_CTLMode=Duty or Period control mode  HRPWM_EDGMode=Both edge  hrpeb=off  enHRPWMB=off  HRPWM_LoadModeB=Counter equals to zero (CTR=ZERO)  HRPWM_CTLModeB=Duty or Period control mode  HRPWM_EDGModeB=Both edge  enHRDBRED=off  enHRDBFED=off  enSFO=on  enautoconv=on  chopperEnable=off  chopperFrequency=1  chopperFirstwidth=1  chopperDuty=12.5%  tripZonesource=Specify via dialog  tzselOSHT1=off  tzselOSHT2=off  tzselOSHT3=off  tzselOSHDCAEV1=off  tzselOSHDCBEV1=off  tzselCBC1=off  tzselCBC2=off  tzselCBC3=off  tzselCBCDCAEV2=off  tzselCBCDCBEV2=off  tzselOSHT4=off  tzselOSHT5=off  tzselOSHT6=off  tzselCBC4=off  tzselCBC5=off  tzselCBC6=off  enTzOstIntr=off  enTzCbcIntr=off  enTzDCAEVT1Intr=off  enTzDCAEVT2Intr=off  enTzDCBEVT1Intr=off  enTzDCBEVT2Intr=off  ePWMxAforced=No action  ePWMxBforced=No action  DCAEVT1forced=No action  DCBEVT1forced=No action  DCAEVT2forced=No action  DCBEVT2forced=No action  dcah=Trip Zone 1 input (TZ1)  dcal=Trip Zone 1 input (TZ1)  dcbh=Trip Zone 1 input (TZ1)  dcbl=Trip Zone 1 input (TZ1)  dcah_type2=GPTRIP1SEL/(TZ1)  dcal_type2=GPTRIP2SEL/(TZ2)  dcbh_type2=GPTRIP1SEL/(TZ1)  dcbl_type2=GPTRIP2SEL/(TZ2)  gendcaevt1=Event disabled  gendcaevt2=Event disabled  gendcbevt1=Event disabled  gendcbevt2=Event disabled  dcaevt1src=DCAEVT1 with sync  dcaevt2src=DCAEVT2 with sync  dcbevt1src=DCBEVT1 with sync  dcbevt2src=DCBEVT2 with sync  pulsesel=Counter equals to zero (CTR=Zero)  blankinv=off  blankoffset=0  blankwidth=0  evsrcsel=Filtered version of DCAEVT1 (DCAEVT1FILT)  encape=off
      settings: LibrarySourceBlock=c2806xlib/ePWM
  wires:
  Prescale Divider/1 -> Divide5/2
  Divide5/1 -> Product2/1, Product3/1, Product1/1, ePWM/1, Display/1, ePWM1/1, ePWM2/1, Product/1
  Product1/1 -> ePWM/2
  EPWMCLK/1 -> Divide4/1
  Gain1/1 -> Divide4/2
  Gain2/1 -> ePWM2/2, ePWM1/2
  Divide6/1 -> Product/2
  Inport/1 -> Gain1/1
  Product2/1 -> ePWM1/3
  Constant3/1 -> Divide6/2
  Inport1/1 -> Divide6/1
  Product3/1 -> ePWM2/3
  Product/1 -> Gain2/1
  Divide4/1 -> Divide5/1
  In2/1 -> Product2/2
  In1/1 -> Product1/2
  In3/1 -> Product3/2
